simulink model "lyapunov_bac_2"  (Simulink 7.3)
settings: Solver=ode5  StartTime=0.0  StopTime=100  FixedStep=0.01  RelTol=1e-3
StopFcn:
  | subplot(211);
  | plot(Data.time,Data.signals(1).values(:,1),'r',Data.time,Data.signals(1).values(:,2),'b')
  | subplot(212);
  | plot(Data.time,Data.signals(2).values(:,1),'b')
libraries: simulink x1
settings Model: Creator=Minh-Map-Vu  LastModifiedBy=nthuy
settings DataIOCC: SignalLoggingName=sigsOut
settings DebuggingCC: SaveWithParameterizedLinksMsg=none  SignalResolutionControl=TryResolveAllWithWarning  SolverPrmCheckMsg=none  MultiTaskDSMMsg=warning  MultiTaskCondExecSysMsg=none  StrictBusMsg=None
settings HardwareCC: TargetEndianess=LittleEndian  TargetHWDeviceType=MATLAB Host  ProdEqTarget=off
settings RTWCC: IncludeERTFirstTime=on

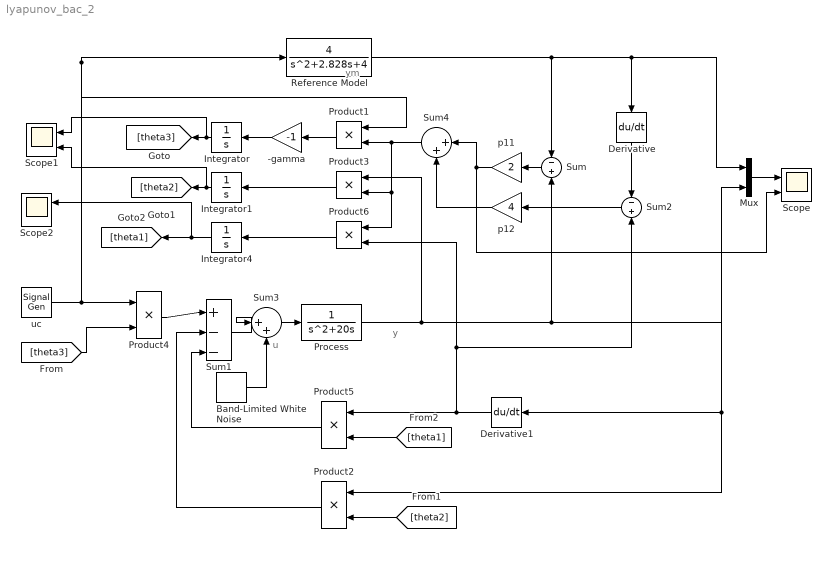
== system lyapunov_bac_2 ==
  note: ym
  note: u
  note: y
  -gamma : Gain  Gain=-1  SaturateOnIntegerOverflow=on  OutDataTypeStr=Inherit: Same as input  ParamDataTypeStr=Inherit: Same as input
  Band-Limited White Noise : simulink/Sources/Band-Limited White Noise  SystemSampleTime=-1  Cov=[.1]  Ts=0.01  seed=[23341]
  Derivative : Derivative
  Derivative1 : Derivative
  Integrator : Integrator
  Integrator1 : Integrator
  Integrator4 : Integrator
  Mux : Mux  Inputs=2
  Process : TransferFcn  Numerator=1  Denominator=[1 20 0]
  Product{1..6} (6 alike) : Product  SaturateOnIntegerOverflow=on  OutDataTypeStr=Inherit: Same as first input
  Reference Model : TransferFcn  Numerator=[4]  Denominator=[1 2.828 4]
  Scope : Scope  NumInputPorts=2
      settings: TimeRange=100  YMin=-1.2~-5  YMax=1.2~5  SaveName=Data
  Scope1 : Scope  NumInputPorts=2
      settings: TimeRange=100  YMin=-1.2~-5  YMax=1.2~5  SaveName=Data1
  Scope2 : Scope  NumInputPorts=2
      settings: TimeRange=100  YMin=-1.2~-5  YMax=1.2~5  SaveName=Data2
  Sum : Sum  Inputs=-+  SaturateOnIntegerOverflow=on
  Sum1 : Sum  Inputs=|+--  SaturateOnIntegerOverflow=on
  Sum2 : Sum  Inputs=-+  SaturateOnIntegerOverflow=on
  Sum3 : Sum  Inputs=|++  SaturateOnIntegerOverflow=on
  Sum4 : Sum  Inputs=|++  SaturateOnIntegerOverflow=on
  p11 : Gain  Gain=2  SaturateOnIntegerOverflow=on  OutDataTypeStr=Inherit: Same as input  ParamDataTypeStr=Inherit: Same as input
  p12 : Gain  Gain=4  SaturateOnIntegerOverflow=on  OutDataTypeStr=Inherit: Same as input  ParamDataTypeStr=Inherit: Same as input
  uc : SignalGenerator  WaveForm=square  Frequency=1/20
  wires:
  uc/1 -> Reference Model/1, Product1/1, Product4/1
  Reference Model/1 -> Sum/1, Mux/1, Derivative/1
  -gamma/1 -> Integrator/1
  Product4/1 -> Sum1/1
  Process/1 -> Mux/2, Product2/1, Derivative1/1, Sum/2, Product3/1
  Product1/1 -> -gamma/1
  Mux/1 -> Scope/1
  Integrator/1 -> Scope1/1, [theta3]
  [theta3] -> Product4/2
  [theta2] -> Product2/2
  Product2/1 -> Sum1/2
  Integrator1/1 -> Scope1/2, [theta2]
  Product3/1 -> Integrator1/1
  [theta1] -> Product5/2
  Derivative1/1 -> Product5/1, Sum2/2, Product6/2
  Product5/1 -> Sum1/3
  Derivative/1 -> Sum2/1
  Sum/1 -> p11/1
  Sum2/1 -> p12/1
  Integrator4/1 -> [theta1], Scope2/1
  Product6/1 -> Integrator4/1
  Sum4/1 -> Product1/2, Product3/2, Product6/1
  p11/1 -> Sum4/1, Scope/2
  p12/1 -> Sum4/2
  Sum1/1 -> Sum3/1
  Band-Limited White Noise/1 -> Sum3/2
  Sum3/1 -> Process/1
